simulink library "lib_gravity"  (R2015a)
settings: Solver=ode45  StartTime=0.0  StopTime=10.0  RelTol=1e-3
undefined symbols (not defined in the file or in its folder): slcm
undefined symbols (not defined in the file): Target
libraries: lib_gravity x2
settings Model: Creator=bbrito  LastModifiedBy=bbrito

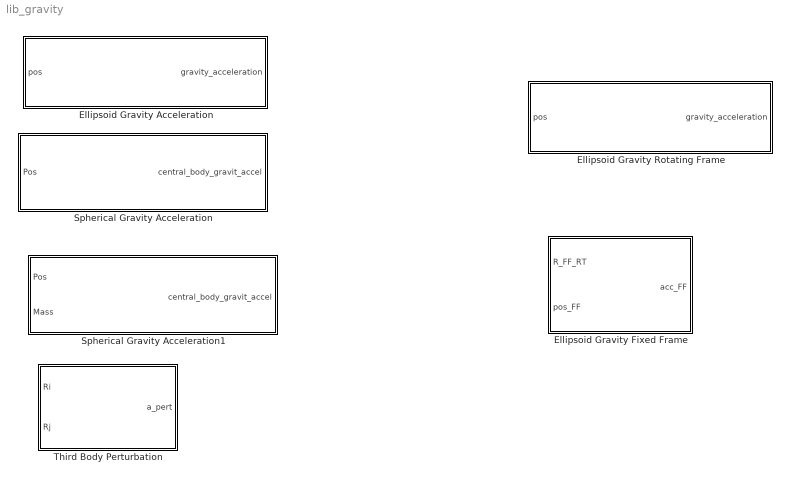
== system lib_gravity ==
  Ellipsoid Gravity Acceleration : MATLAB Function  TreatAsAtomicUnit=on  mask{dim=Target.ModelData.Secondary.dim, r0=Target.ModelData.r0, u=Target.ModelData.GravitationalConstant}
      mask prompts: dim "Ellipsoid Dimensions"; r0 "Normalized Distance"; u "Gravitational Constant"
      mask help:
      | ESA-ESTEC
      | ---------------------------------------------------------------------------
      | Version:0.1          Date:4/11/20015          Author: #BB
      | Matlab version: 2015a          Project: AIM          Division: TEC-ECN
      | ---------------------------------------------------------------------------
      | This block models the ellipsoid model gravity acceleration.
      |
      | The input is the x,y,z relative to the center of mass of the body, in the ellisoid body frame.
      |
      | The model reference can be found in:
  Ellipsoid Gravity Fixed Frame : Subsystem  TreatAsAtomicUnit=on  mask{dim=[0;0;0], r0=0, u=0}
      mask prompts: dim "Ellipsoid dimensions"; r0 "Normalized distance"; u "Gravitational constant"
      mask help:
      | ESA-ESTEC
      | ---------------------------------------------------------------------------
      | Version:0.0          Date:8/10/20015          Author: #BB
      | Matlab version: 2015a          Project: AIM          Division: TEC-ECN
      | ---------------------------------------------------------------------------
      | This block models the shperical central body gravitation acceleration.
      |
      | The input is the x,y,z relative to the center of mass of the body in Fixed Frame (FF).
      |     The matrix R_FF_RT will rotate the position coordinates in Fixed Frame to the Rotating Frame (RT) of the ellipsoid. The rotating frame is fixed to the body of the ellipsoid.
      | The parameter r0 is the average or the maximum radius  of the ellipsoid.
      |
      | The ellipsoid dimensions is the vector [alfa;beta;gama] as represented in the picture.
      |
      | Reference: Orbital Motion in Strongly Perturbed Environments
      | Authors: Scheeres, Daniel J.
  Ellipsoid Gravity Rotating Frame : MATLAB Function  TreatAsAtomicUnit=on  mask{dim=Target.ModelData.Secondary.dim, r0=Target.ModelData.r0, u=Target.ModelData.GravitationalConstant}
      mask prompts: dim "Ellipsoid Dimensions"; r0 "Normalized Distance"; u "Gravitational Constant"
      mask help:
      | ESA-ESTEC
      | ---------------------------------------------------------------------------
      | Version:0.0          Date:8/10/20015          Author: #BB
      | Matlab version: 2015a          Project: AIM          Division: TEC-ECN
      | ---------------------------------------------------------------------------
      | This block models the shperical central body gravitation acceleration.
      |
      | The input is the x,y,z relative to the center of mass of the body.
      |
      | The parameter r0 is the average or the maximum radius  of the ellipsoid.
      |
      | The ellipsoid dimensions is the vector [alfa;beta;gama] as represented in the picture.
      |
      | Reference: Orbital Motion in Strongly Perturbed Environments
      | Authors: Scheeres, Daniel J.
  Spherical Gravity Acceleration : Subsystem  TreatAsAtomicUnit=on  mask{u=Target.ModelData.Secondary.GravitationalConstant2}
      mask prompts: u "Target Gravitational Constant"
      mask help:
      | ESA-ESTEC
      | ---------------------------------------------------------------------------
      | Version:0.0          Date:8/10/20015          Author: #BB
      | Matlab version: 2015a          Project: AIM          Division: TEC-ECN
      | ---------------------------------------------------------------------------
      | This block models the shperical central body gravitation acceleration.
      |
      | The input is the x,y,z relative to the center of mass of the body.
  Spherical Gravity Acceleration1 : Subsystem  AncestorBlock=lib_gravity/Spherical Gravity Acceleration  TreatAsAtomicUnit=on  mask{u=0}
      mask prompts: u "Gravitational constant"
      mask help:
      | ESA-ESTEC
      | ---------------------------------------------------------------------------
      | Version:0.0          Date:13/10/20015          Author: #BB
      | Matlab version: 2015a          Project: AIM          Division: TEC-ECN
      | ---------------------------------------------------------------------------
      | This block models the shperical central body gravitation acceleration.
      |
      | The input is the x,y,z relative to the center of mass of the body.
  Third Body Perturbation : Subsystem  TreatAsAtomicUnit=on  mask{u=0}
      mask prompts: u "Gravitational constant"
      mask help:
      | ESA-ESTEC
      | ---------------------------------------------------------------------------
      | Version:0.0          Date:8/10/20015          Author: #BB
      | Matlab version: 2015a          Project: AIM          Division: TEC-ECN
      | ---------------------------------------------------------------------------
      | This block models the shperical central body gravitation perturbation acceleration.
      |
      | The input is the perturbing body vector position Rj in cartesian coordinates.
      |
      | Ri is the point mass position vector in cartesian coordinates that is being perturbed.

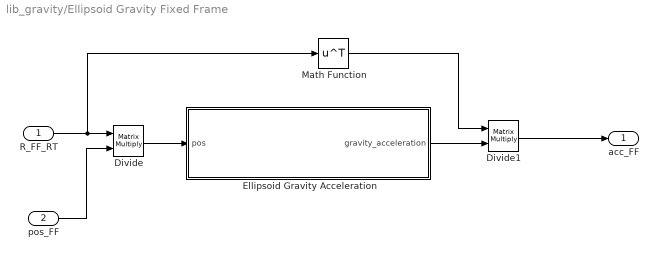
== system lib_gravity/Ellipsoid Gravity Fixed Frame ==
  R_FF_RT : Inport
  pos_FF : Inport  Port=2
  Divide : Product  Inputs=**  Multiplication=Matrix(*)
  Divide1 : Product  Inputs=**  Multiplication=Matrix(*)
  Ellipsoid Gravity Acceleration : MATLAB Function  TreatAsAtomicUnit=on
  Math Function : Math  Operator=transpose  SaturateOnIntegerOverflow=on
  acc_FF : Outport
  wires:
  R_FF_RT/1 -> Math Function/1, Divide/1
  Math Function/1 -> Divide1/1
  Ellipsoid Gravity Acceleration/1(gravity_acceleration) -> Divide1/2
  Divide/1 -> Ellipsoid Gravity Acceleration/1(pos)
  pos_FF/1 -> Divide/2
  Divide1/1 -> acc_FF/1

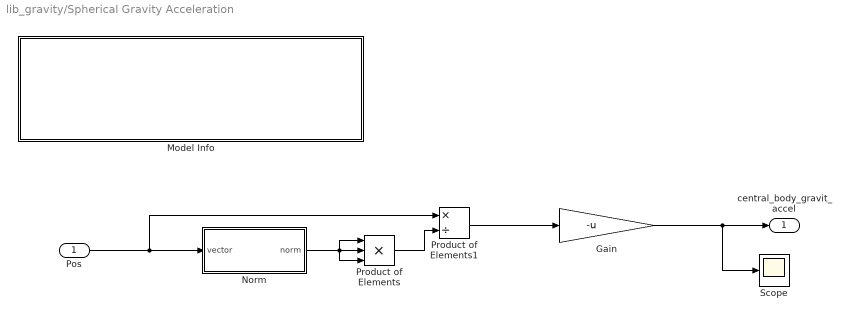
== system lib_gravity/Spherical Gravity Acceleration ==
  Pos : Inport
  Gain : Gain  Gain=-u
  Model Info : Subsystem  LoadFcn=slcm LoadBlock;  InitFcn=slcm('UpdateAllCMBlocksInThisModelInit')  mask(CMBlock){InitialSaveTempField=, InitialBlockCM=, BlockCM=, Frame=on, SaveTempField=, DisplayStringWithTags=|, MaskDisplayString=ESA-ESTEC\n---------------------------------------------------------------------------\nVersion:0.0          Date:8/10/20015          Author: #BB\nMatlab version: 2015a          Project: AIM          Division: TEC-ECN\n---------------------------------------------------------------------------\nThis block models the shperical central body gravitation acceleration.\n\nThe input is the x,y,z relative to the center of mass of the body., HorizontalTextAlignment=Center, LeftAlignmentValue=0.5, SourceBlockDiagram=AIM_v0, TagMaxNumber=20, CMTag1=, CMTag2=, CMTag3=, CMTag4=, CMTag5=, CMTag6=, CMTag7=, CMTag8=, CMTag9=, CMTag10=, CMTag11=, CMTag12=, CMTag13=, CMTag14=, CMTag15=, CMTag16=, CMTag17=, CMTag18=, CMTag19=, CMTag20=}
      mask DisplayStringWithTags=|
      | ESA-ESTEC
      | ---------------------------------------------------------------------------
      | Version:0.0          Date:8/10/20015          Author: #BB
      | Matlab version: 2015a          Project: AIM          Division: TEC-ECN
      | ---------------------------------------------------------------------------
      | This block models the shperical central body gravitation acceleration.
      |
      | The input is the x,y,z relative to the center of mass of the body.
      mask help: This block allows revision control information to be displayed within the model.
      settings: CopyFcn=slcm CopyBlock;  DeleteFcn=slcm Cancel;  PostSaveFcn=slcm('UpdateAllCMBlocksInThisModel')  NameChangeFcn=slcm Rename;  OpenFcn=slcm
      mask Display: text(str2num(LeftAlignmentValue), 0.5, MaskDisplayString, 'HorizontalAlignment', HorizontalTextAlignment)
  Norm : Subsystem
  Product of Elements : Product  Inputs=***
  Product of Elements1 : Product  Inputs=*/
  Scope : Scope
      settings: YMin=-5.5e-05  YMax=3e-05  SaveName=ScopeData9
  central_body_gravit_accel : Outport
  wires:
  Norm/1(norm) -> Product of Elements/3, Product of Elements/1, Product of Elements/2
  Product of Elements/1 -> Product of Elements1/2
  Gain/1 -> central_body_gravit_accel/1, Scope/1
  Product of Elements1/1 -> Gain/1
  Pos/1 -> Product of Elements1/1, Norm/1(vector)

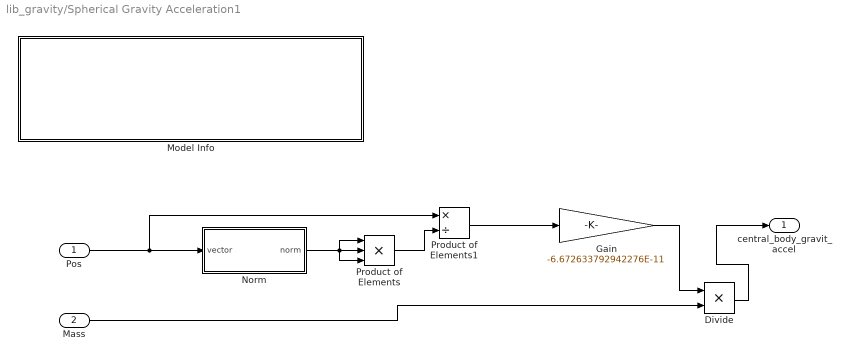
== system lib_gravity/Spherical Gravity Acceleration1 ==
  Pos : Inport
  Mass : Inport  Port=2
  Divide : Product  Inputs=**
  Gain : Gain  Gain=-6.672633792942276E-11
  Model Info : Subsystem  LoadFcn=slcm LoadBlock;  InitFcn=slcm('UpdateAllCMBlocksInThisModelInit')  mask(CMBlock){InitialSaveTempField=, InitialBlockCM=, BlockCM=, Frame=on, SaveTempField=, DisplayStringWithTags=|, MaskDisplayString=ESA-ESTEC\n---------------------------------------------------------------------------\nVersion:0.0          Date:8/10/20015          Author: #BB\nMatlab version: 2015a          Project: AIM          Division: TEC-ECN\n---------------------------------------------------------------------------\nThis block models the shperical central body gravitation acceleration.\n\nThe input is the x,y,z relative to the center of mass of the body., HorizontalTextAlignment=Center, LeftAlignmentValue=0.5, SourceBlockDiagram=lib_gravity, TagMaxNumber=20, CMTag1=, CMTag2=, CMTag3=, CMTag4=, CMTag5=, CMTag6=, CMTag7=, CMTag8=, CMTag9=, CMTag10=, CMTag11=, CMTag12=, CMTag13=, CMTag14=, CMTag15=, CMTag16=, CMTag17=, CMTag18=, CMTag19=, CMTag20=}
      mask DisplayStringWithTags=|
      | ESA-ESTEC
      | ---------------------------------------------------------------------------
      | Version:0.0          Date:8/10/20015          Author: #BB
      | Matlab version: 2015a          Project: AIM          Division: TEC-ECN
      | ---------------------------------------------------------------------------
      | This block models the shperical central body gravitation acceleration.
      |
      | The input is the x,y,z relative to the center of mass of the body.
      mask help: This block allows revision control information to be displayed within the model.
      settings: CopyFcn=slcm CopyBlock;  DeleteFcn=slcm Cancel;  PostSaveFcn=slcm('UpdateAllCMBlocksInThisModel')  NameChangeFcn=slcm Rename;  OpenFcn=slcm
      mask Display: text(str2num(LeftAlignmentValue), 0.5, MaskDisplayString, 'HorizontalAlignment', HorizontalTextAlignment)
  Norm : Subsystem
  Product of Elements : Product  Inputs=***
  Product of Elements1 : Product  Inputs=*/
  central_body_gravit_accel : Outport
  wires:
  Norm/1(norm) -> Product of Elements/3, Product of Elements/1, Product of Elements/2
  Product of Elements/1 -> Product of Elements1/2
  Product of Elements1/1 -> Gain/1
  Pos/1 -> Product of Elements1/1, Norm/1(vector)
  Gain/1 -> Divide/1
  Mass/1 -> Divide/2
  Divide/1 -> central_body_gravit_accel/1

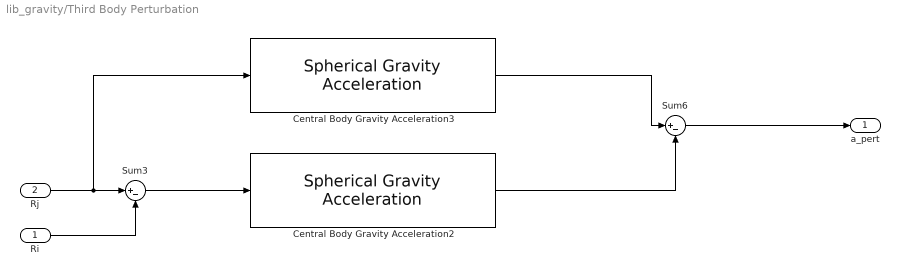
== system lib_gravity/Third Body Perturbation ==
  Ri : Inport
  Rj : Inport  Port=2
  Central Body Gravity Acceleration2 : lib_gravity/Spherical Gravity Acceleration  u=u
  Central Body Gravity Acceleration3 : lib_gravity/Spherical Gravity Acceleration  u=u
  Sum3 : Sum  Inputs=|+-
  Sum6 : Sum  Inputs=|+-
  a_pert : Outport
  wires:
  Central Body Gravity Acceleration3/1 -> Sum6/1
  Central Body Gravity Acceleration2/1 -> Sum6/2
  Sum3/1 -> Central Body Gravity Acceleration2/1
  Ri/1 -> Sum3/2
  Rj/1 -> Central Body Gravity Acceleration3/1, Sum3/1
  Sum6/1 -> a_pert/1

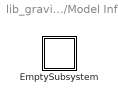
== system lib_gravity/Spherical Gravity Acceleration/Model Info ==
  EmptySubsystem : Subsystem

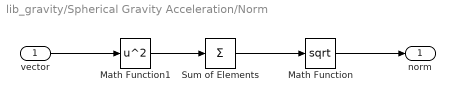
== system lib_gravity/Spherical Gravity Acceleration/Norm ==
  vector : Inport
  Math Function : Math  Operator=sqrt  SaturateOnIntegerOverflow=on
  Math Function1 : Math  Operator=square  SaturateOnIntegerOverflow=on
  Sum of Elements : Sum  Inputs=+
  norm : Outport
  wires:
  Sum of Elements/1 -> Math Function/1
  Math Function1/1 -> Sum of Elements/1
  vector/1 -> Math Function1/1
  Math Function/1 -> norm/1

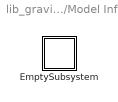
== system lib_gravity/Spherical Gravity Acceleration1/Model Info ==
  EmptySubsystem : Subsystem

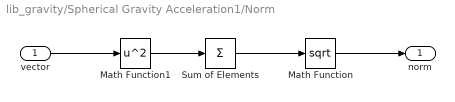
== system lib_gravity/Spherical Gravity Acceleration1/Norm ==
  vector : Inport
  Math Function : Math  Operator=sqrt  SaturateOnIntegerOverflow=on
  Math Function1 : Math  Operator=square  SaturateOnIntegerOverflow=on
  Sum of Elements : Sum  Inputs=+
  norm : Outport
  wires:
  Sum of Elements/1 -> Math Function/1
  Math Function1/1 -> Sum of Elements/1
  vector/1 -> Math Function1/1
  Math Function/1 -> norm/1

== system lib_gravity/Spherical Gravity Acceleration/Model Info/EmptySubsystem ==

== system lib_gravity/Spherical Gravity Acceleration1/Model Info/EmptySubsystem ==

== matlab function lib_gravity/Ellipsoid Gravity Acceleration ==
  data: pos input; gravity_acceleration output; dim parameter; r0 parameter; u parameter
function gravity_acceleration = fcn(pos, dim, r0, u)


alfa=dim(1);
gama=dim(2);
beta=dim(3);

x=pos(1);
y=pos(2);
z=pos(3);

%Gravitational coeficients
c20 = 1/(5*r0^2)*(gama^2-(alfa^2+beta^2)/2);
c22 = 1/(20*r0^2)*(alfa^2-beta^2);
c40 = 15/7*(c20^2+2*c22^2);
c42 = 5/7*c20*c22;
c44 = 5/28*c22^2;

%Gravitational parameter of the body

%Spherical coordinates

r=sqrt(x^2+y^2+z^2);
delta=asin(z/r);
lambda=atan2(y,x);


%Associated legendre functions
%Necessary to intialize varibles because of extrinsic function
P20 = 0;%0.5*(3*sin(delta)^2-1);
P21 = 0;%3*sin(delta)*sqrt((1-sin(delta)^2));
P22 = 0;%3*(1-sin(delta)^2);
P40 = 0;%1/8*(35*sin(delta)^4-30*sin(delta)^2+3);
P41 = 0;%5/2*(7*sin(delta)^3-3*sin(delta))*sqrt(1-sin(delta)^2);
P42 = 0;%15/2*(7*sin(delta)^2-1)*(1-sin(delta)^2);
P43 = 0;%105*sin(delta)*(sqrt((1-sin(delta)^2))^3);
P44 = 0;%105*(1-sin(delta)^2)^2;

P20 = 0.5*(3*sin(delta)^2-1);
P21 = 3*sin(delta)*sqrt((1-sin(delta)^2));
P22 = 3*(1-sin(delta)^2);
P40 = 1/8*(35*sin(delta)^4-30*sin(delta)^2+3);
P41 = 5/2*(7*sin(delta)^3-3*sin(delta))*sqrt(1-sin(delta)^2);
P42 = 15/2*(7*sin(delta)^2-1)*(1-sin(delta)^2);
P43 = 105*sin(delta)*(sqrt((1-sin(delta)^2))^3);
P44 = 105*(1-sin(delta)^2)^2;


%Potencial calculation

grav_gradient_r=-(u/(r^2))*(1+3*((r0/r)^2)*P20*c20 + c22*3*((r0/r)^2)*P22*cos(2*lambda) + c40*5*((r0/r)^4)*P40 + c42*5*((r0/r)^4)*P42*cos(2*lambda)+c44*5*((r0/r)^4)*P44*cos(4*lambda));


grav_gradient_delta=(u/r)* ((r0/r)^2*(P21*c20-2*tan(delta)*P22*c22*cos(2*lambda)) + (r0/r)^4*(P41*c40+(P43-2*tan(delta)*P42)*c42*cos(2*lambda)-4*tan(delta)*P44*c44*cos(4*lambda)));



grav_gradient_lambda=-(u/r)*((r0/r)^2*2*P22*c22*sin(2*lambda)+(r0/r)^4*2*P42*c42*sin(2*lambda)+(r0/r)^4*4*P44*c44*sin(4*lambda));



grav_gradient_x=cos(delta)*cos(lambda)*grav_gradient_r-(sin(delta)*cos(lambda))/r*grav_gradient_delta-sin(lambda)/cos(delta)/r*grav_gradient_lambda;

grav_gradient_y=cos(delta)*sin(lambda)*grav_gradient_r-(sin(delta)*sin(lambda))/r*grav_gradient_delta-cos(lambda)/cos(delta)/r*grav_gradient_lambda;

grav_gradient_z=sin(delta)*grav_gradient_r-cos(delta)/r*grav_gradient_delta;


gravity_acceleration = [grav_gradient_x;grav_gradient_y;grav_gradient_z];

== matlab function lib_gravity/Ellipsoid Gravity Fixed Frame/Ellipsoid Gravity Acceleration ==
  data: pos input; gravity_acceleration output; dim parameter; r0 parameter; u parameter
function gravity_acceleration = fcn(pos, dim, r0, u)


alfa=dim(1);
gama=dim(2);
beta=dim(3);

x=pos(1);
y=pos(2);
z=pos(3);

%Gravitational coeficients
c20 = 1/(5*r0^2)*(gama^2-(alfa^2+beta^2)/2);
c22 = 1/(20*r0^2)*(alfa^2-beta^2);
c40 = 15/7*(c20^2+2*c22^2);
c42 = 5/7*c20*c22;
c44 = 5/28*c22^2;

%Gravitational parameter of the body

%Spherical coordinates

r=sqrt(x^2+y^2+z^2);
delta=asin(z/r);
lambda=atan2(y,x);


%Associated legendre functions
%Necessary to intialize varibles because of extrinsic function
P20 = 0;%0.5*(3*sin(delta)^2-1);
P21 = 0;%3*sin(delta)*sqrt((1-sin(delta)^2));
P22 = 0;%3*(1-sin(delta)^2);
P40 = 0;%1/8*(35*sin(delta)^4-30*sin(delta)^2+3);
P41 = 0;%5/2*(7*sin(delta)^3-3*sin(delta))*sqrt(1-sin(delta)^2);
P42 = 0;%15/2*(7*sin(delta)^2-1)*(1-sin(delta)^2);
P43 = 0;%105*sin(delta)*(sqrt((1-sin(delta)^2))^3);
P44 = 0;%105*(1-sin(delta)^2)^2;

P20 = 0.5*(3*sin(delta)^2-1);
P21 = 3*sin(delta)*sqrt((1-sin(delta)^2));
P22 = 3*(1-sin(delta)^2);
P40 = 1/8*(35*sin(delta)^4-30*sin(delta)^2+3);
P41 = 5/2*(7*sin(delta)^3-3*sin(delta))*sqrt(1-sin(delta)^2);
P42 = 15/2*(7*sin(delta)^2-1)*(1-sin(delta)^2);
P43 = 105*sin(delta)*(sqrt((1-sin(delta)^2))^3);
P44 = 105*(1-sin(delta)^2)^2;


%Potencial calculation

grav_gradient_r=-(u/(r^2))*(1+3*((r0/r)^2)*P20*c20 + c22*3*((r0/r)^2)*P22*cos(2*lambda) + c40*5*((r0/r)^4)*P40 + c42*5*((r0/r)^4)*P42*cos(2*lambda)+c44*5*((r0/r)^4)*P44*cos(4*lambda));


grav_gradient_delta=(u/r)* ((r0/r)^2*(P21*c20-2*tan(delta)*P22*c22*cos(2*lambda)) + (r0/r)^4*(P41*c40+(P43-2*tan(delta)*P42)*c42*cos(2*lambda)-4*tan(delta)*P44*c44*cos(4*lambda)));



grav_gradient_lambda=-(u/r)*((r0/r)^2*2*P22*c22*sin(2*lambda)+(r0/r)^4*2*P42*c42*sin(2*lambda)+(r0/r)^4*4*P44*c44*sin(4*lambda));



grav_gradient_x=cos(delta)*cos(lambda)*grav_gradient_r-(sin(delta)*cos(lambda))/r*grav_gradient_delta-sin(lambda)/cos(delta)/r*grav_gradient_lambda;

grav_gradient_y=cos(delta)*sin(lambda)*grav_gradient_r-(sin(delta)*sin(lambda))/r*grav_gradient_delta-cos(lambda)/cos(delta)/r*grav_gradient_lambda;

grav_gradient_z=sin(delta)*grav_gradient_r-cos(delta)/r*grav_gradient_delta;


gravity_acceleration = [grav_gradient_x;grav_gradient_y;grav_gradient_z];

== matlab function lib_gravity/Ellipsoid Gravity Rotating Frame ==
  data: pos input; gravity_acceleration output; dim parameter; r0 parameter; u parameter
function gravity_acceleration = fcn(pos, dim, r0, u)


alfa=dim(1);
gama=dim(2);
beta=dim(3);

x=pos(1);
y=pos(2);
z=pos(3);

%Gravitational coeficients
c20 = 1/(5*r0^2)*(gama^2-(alfa^2+beta^2)/2);
c22 = 1/(20*r0^2)*(alfa^2-beta^2);
c40 = 15/7*(c20^2+2*c22^2);
c42 = 5/7*c20*c22;
c44 = 5/28*c22^2;

%Gravitational parameter of the body

%Spherical coordinates

r=sqrt(x^2+y^2+z^2);
delta=asin(z/r);
lambda=atan2(y,x);


%Associated legendre functions
%Necessary to intialize varibles because of extrinsic function

P20 = 0;%0.5*(3*sin(delta)^2-1);
P21 = 0;%3*sin(delta)*sqrt((1-sin(delta)^2));
P22 = 0;%3*(1-sin(delta)^2);
P40 = 0;%1/8*(35*sin(delta)^4-30*sin(delta)^2+3);
P41 = 0;%5/2*(7*sin(delta)^3-3*sin(delta))*sqrt(1-sin(delta)^2);
P42 = 0;%15/2*(7*sin(delta)^2-1)*(1-sin(delta)^2);
P43 = 0;%105*sin(delta)*(sqrt((1-sin(delta)^2))^3);
P44 = 0;%105*(1-sin(delta)^2)^2;

P20 = 0.5*(3*sin(delta)^2-1);
P21 = 3*sin(delta)*sqrt((1-sin(delta)^2));
P22 = 3*(1-sin(delta)^2);
P40 = 1/8*(35*sin(delta)^4-30*sin(delta)^2+3);
P41 = 5/2*(7*sin(delta)^3-3*sin(delta))*sqrt(1-sin(delta)^2);
P42 = 15/2*(7*sin(delta)^2-1)*(1-sin(delta)^2);
P43 = 105*sin(delta)*(sqrt((1-sin(delta)^2))^3);
P44 = 105*(1-sin(delta)^2)^2;

%Potencial calculation

grav_gradient_r=-(u/(r^2))*(1+3*((r0/r)^2)*P20*c20 + c22*3*((r0/r)^2)*P22*cos(2*lambda) + c40*5*((r0/r)^4)*P40 + c42*5*((r0/r)^4)*P42*cos(2*lambda)+c44*5*((r0/r)^4)*P44*cos(4*lambda));


grav_gradient_delta=(u/r)* ((r0/r)^2*(P21*c20-2*tan(delta)*P22*c22*cos(2*lambda)) + (r0/r)^4*(P41*c40+(P43-2*tan(delta)*P42)*c42*cos(2*lambda)-4*tan(delta)*P44*c44*cos(4*lambda)));



grav_gradient_lambda=-(u/r)*((r0/r)^2*2*P22*c22*sin(2*lambda)+(r0/r)^4*2*P42*c42*sin(2*lambda)+(r0/r)^4*4*P44*c44*sin(4*lambda));



grav_gradient_x=cos(delta)*cos(lambda)*grav_gradient_r-(sin(delta)*cos(lambda))/r*grav_gradient_delta-sin(lambda)/cos(delta)/r*grav_gradient_lambda;

grav_gradient_y=cos(delta)*sin(lambda)*grav_gradient_r-(sin(delta)*sin(lambda))/r*grav_gradient_delta-cos(lambda)/cos(delta)/r*grav_gradient_lambda;

grav_gradient_z=sin(delta)*grav_gradient_r-cos(delta)/r*grav_gradient_delta;

%  H=inv([cos(delta)*cos(lambda) cos(delta)*sin(lambda) sin(delta);-sin(lambda) cos(lambda) 0;-sin(delta)*cos(lambda) -sin(delta)*sin(lambda) cos(delta)]);
%  
% grav=H*[grav_gradient_r;grav_gradient_delta;grav_gradient_lambda];
% 
% grav_gradient_x=grav(1);
% grav_gradient_y=grav(2);
% grav_gradient_z=grav(3);

gravity_acceleration = [grav_gradient_x;grav_gradient_y;grav_gradient_z];
